simulink model "UG_model"  (R2024b)
settings: Solver=VariableStepAuto  StartTime=0.0  StopTime=500  FixedStep=0.0001  RelTol=1e-3
settings Model: Creator=yang1118  LastModifiedBy=leste
settings RTWCC: GPUComputeCapability=3.5

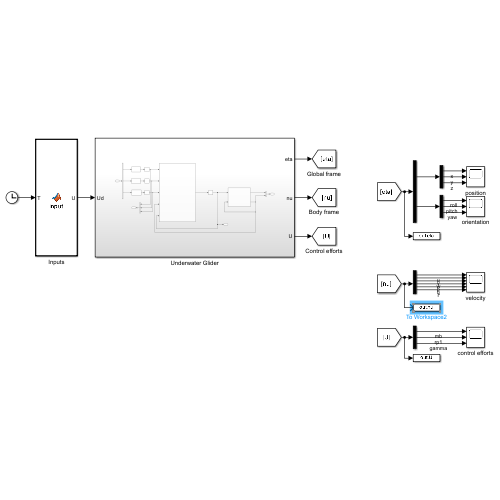
[thumbnail: Simulink's stored preview of the top-level diagram]
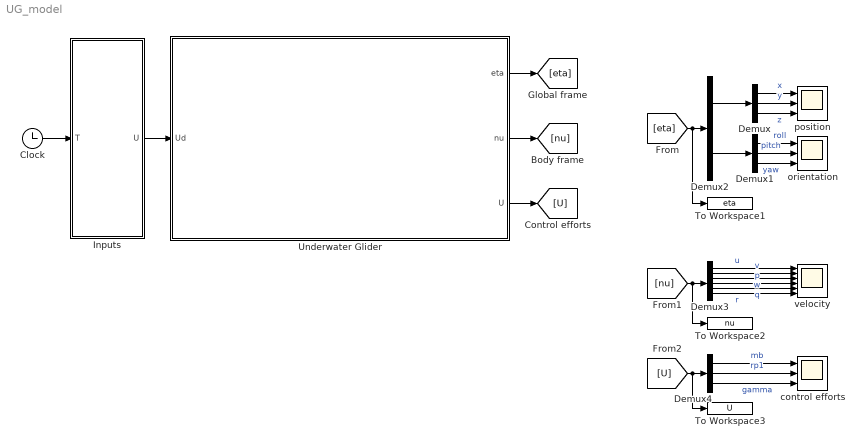
== system UG_model ==
  Clock : Clock
  Demux : Demux  Outputs=3
  Demux1 : Demux  Outputs=3
  Demux2 : Demux  Outputs=2
  Demux3 : Demux  Outputs=6
  Demux4 : Demux  Outputs=3
  Inputs : MATLAB Function  TreatAsAtomicUnit=on
  To Workspace1 : ToWorkspace  VariableName=eta  SampleTime=-1
      settings: Save2DSignal=2-D array (concatenate along first dimension)
  To Workspace2 : ToWorkspace  VariableName=nu  SampleTime=-1
      settings: Save2DSignal=2-D array (concatenate along first dimension)
  To Workspace3 : ToWorkspace  VariableName=U  SampleTime=-1
      settings: Save2DSignal=2-D array (concatenate along first dimension)
  Underwater Glider : Subsystem
  control efforts : Scope  NumInputPorts=3
  orientation : Scope  NumInputPorts=3
  position : Scope  NumInputPorts=3
  velocity : Scope  NumInputPorts=6
  wires:
  Clock/1 -> Inputs/1(T)
  Demux/1 -> position/1  "x"
  Demux/2 -> position/2  "y"
  Demux/3 -> position/3  "z"
  Demux1/1 -> orientation/1  "roll"
  Demux1/2 -> orientation/2  "pitch"
  Demux1/3 -> orientation/3  "yaw"
  Demux2/1 -> Demux/1
  Demux2/2 -> Demux1/1
  Demux3/5 -> velocity/5  "q"
  Demux3/6 -> velocity/6  "r"
  Demux3/2 -> velocity/2  "v"
  Demux3/1 -> velocity/1  "u"
  Demux3/3 -> velocity/3  "w"
  Demux3/4 -> velocity/4  "p"
  Inputs/1(U) -> Underwater Glider/1(Ud)
  Underwater Glider/1(eta) -> [eta]
  Underwater Glider/2(nu) -> [nu]
  Underwater Glider/3(U) -> [U]
  [eta] -> To Workspace1/1, Demux2/1
  [nu] -> To Workspace2/1, Demux3/1
  [U] -> To Workspace3/1, Demux4/1
  Demux4/1 -> control efforts/1  "mb"
  Demux4/2 -> control efforts/2  "rp1"
  Demux4/3 -> control efforts/3  "gamma"

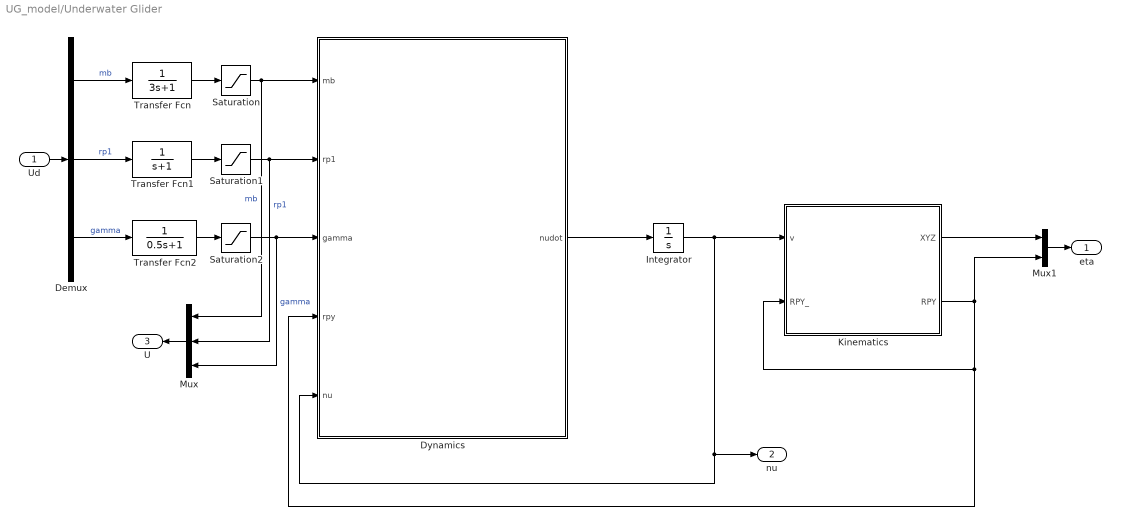
== system UG_model/Underwater Glider ==
  Ud : Inport
  Demux : Demux  Outputs=3
  Dynamics : MATLAB Function  TreatAsAtomicUnit=on
  Integrator : Integrator
  Kinematics : Subsystem
  Mux : Mux  Inputs=3
  Mux1 : Mux  Inputs=2
  Saturation : Saturate  UpperLimit=0.4  LowerLimit=-0.4
  Saturation1 : Saturate  UpperLimit=0.06  LowerLimit=-0.06
  Saturation2 : Saturate  UpperLimit=pi/2  LowerLimit=-pi/2
  Transfer Fcn : TransferFcn  Denominator=[3 1]
  Transfer Fcn1 : TransferFcn  Denominator=[1 1]
  Transfer Fcn2 : TransferFcn  Denominator=[0.5 1]
  eta : Outport
  nu : Outport  Port=2
  U : Outport  Port=3
  wires:
  Kinematics/2(RPY) -> Mux1/2, Kinematics/2(RPY_), Dynamics/4(rpy)
  Saturation/1 -> Mux/1, Dynamics/1(mb)  "mb"
  Saturation1/1 -> Dynamics/2(rp1), Mux/2  "rp1"
  Saturation2/1 -> Dynamics/3(gamma), Mux/3  "gamma"
  Dynamics/1(nudot) -> Integrator/1
  Integrator/1 -> nu/1, Dynamics/5(nu), Kinematics/1(v)
  Mux/1 -> U/1
  Transfer Fcn/1 -> Saturation/1
  Transfer Fcn1/1 -> Saturation1/1
  Transfer Fcn2/1 -> Saturation2/1
  Kinematics/1(XYZ) -> Mux1/1
  Mux1/1 -> eta/1
  Ud/1 -> Demux/1
  Demux/1 -> Transfer Fcn/1  "mb"
  Demux/2 -> Transfer Fcn1/1  "rp1"
  Demux/3 -> Transfer Fcn2/1  "gamma"

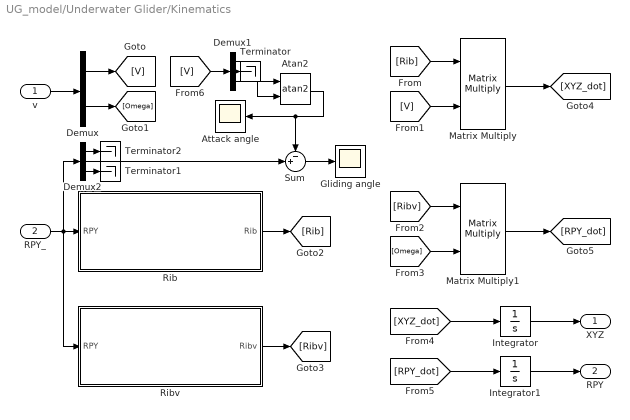
== system UG_model/Underwater Glider/Kinematics ==
  v : Inport  PortDimensions=[6,1]
  RPY_ : Inport  Port=2
  Atan2 : Trigonometry  Operator=atan2
  Attack angle : Scope
  Demux : Demux  Outputs=2
  Demux1 : Demux  Outputs=3
  Demux2 : Demux  Outputs=3
  Gliding angle : Scope
  Integrator : Integrator
  Integrator1 : Integrator
  Matrix Multiply : Product  Multiplication=Matrix(*)
  Matrix Multiply1 : Product  Multiplication=Matrix(*)
  Rib : Subsystem
  Ribv : Subsystem
  Sum : Sum  Inputs=-+|
  Terminator : Terminator
  Terminator1 : Terminator
  Terminator2 : Terminator
  XYZ : Outport
  RPY : Outport  Port=2
  wires:
  v/1 -> Demux/1
  Demux/1 -> [V]
  Demux/2 -> [Omega]
  RPY_/1 -> Demux2/1, Ribv/1(RPY), Rib/1(RPY)
  Rib/1(Rib) -> [Rib]
  Ribv/1(Ribv) -> [Ribv]
  [Rib] -> Matrix Multiply/1
  [V] -> Matrix Multiply/2
  Matrix Multiply/1 -> [XYZ_dot]
  [Ribv] -> Matrix Multiply1/1
  [Omega] -> Matrix Multiply1/2
  Matrix Multiply1/1 -> [RPY_dot]
  Integrator/1 -> XYZ/1
  Integrator1/1 -> RPY/1
  [XYZ_dot] -> Integrator/1
  [RPY_dot] -> Integrator1/1
  [V] -> Demux1/1
  Demux1/2 -> Terminator/1
  Demux1/3 -> Atan2/1
  Demux1/1 -> Atan2/2
  Demux2/3 -> Terminator1/1
  Demux2/1 -> Terminator2/1
  Sum/1 -> Gliding angle/1
  Demux2/2 -> Sum/2
  Atan2/1 -> Sum/1, Attack angle/1

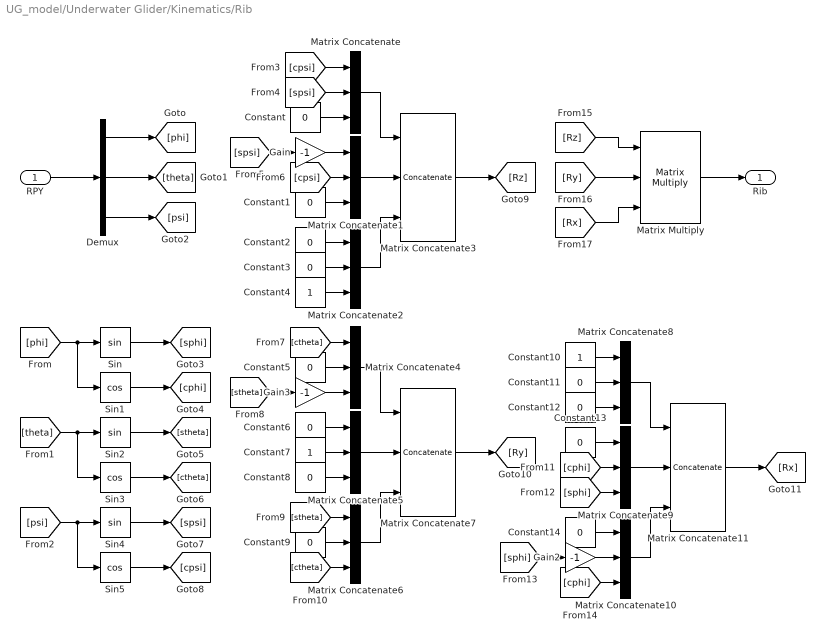
== system UG_model/Underwater Glider/Kinematics/Rib ==
  RPY : Inport  PortDimensions=[3,1]
  Constant{,1..3,5..6,8..9,11..14} (12 alike) : Constant  Value=0
  Constant10 : Constant
  Constant4 : Constant
  Constant7 : Constant
  Demux : Demux  Outputs=3
  Gain : Gain  Gain=-1
  Gain2 : Gain  Gain=-1
  Gain3 : Gain  Gain=-1
  Matrix Concatenate{,1..2,4..6,8..10} (9 alike) : Concatenate  NumInputs=3  ConcatenateDimension=2
  Matrix Concatenate11 : Concatenate  NumInputs=3  Mode=Multidimensional array  ConcatenateDimension=2
  Matrix Concatenate3 : Concatenate  NumInputs=3  Mode=Multidimensional array  ConcatenateDimension=2
  Matrix Concatenate7 : Concatenate  NumInputs=3  Mode=Multidimensional array  ConcatenateDimension=2
  Matrix Multiply : Product  Inputs=3  Multiplication=Matrix(*)
  Sin : Trigonometry
  Sin1 : Trigonometry  Operator=cos
  Sin2 : Trigonometry
  Sin3 : Trigonometry  Operator=cos
  Sin4 : Trigonometry
  Sin5 : Trigonometry  Operator=cos
  Rib : Outport  PortDimensions=[3,3]
  wires:
  Demux/3 -> [psi]
  Demux/1 -> [phi]
  Demux/2 -> [theta]
  RPY/1 -> Demux/1
  [phi] -> Sin1/1, Sin/1
  [theta] -> Sin2/1, Sin3/1
  [psi] -> Sin5/1, Sin4/1
  Sin/1 -> [sphi]
  Sin1/1 -> [cphi]
  Sin2/1 -> [stheta]
  Sin3/1 -> [ctheta]
  Sin4/1 -> [spsi]
  Sin5/1 -> [cpsi]
  [cpsi] -> Matrix Concatenate/1
  [spsi] -> Matrix Concatenate/2
  Constant/1 -> Matrix Concatenate/3
  Gain/1 -> Matrix Concatenate1/1
  [spsi] -> Gain/1
  [cpsi] -> Matrix Concatenate1/2
  Constant1/1 -> Matrix Concatenate1/3
  Constant2/1 -> Matrix Concatenate2/1
  Constant3/1 -> Matrix Concatenate2/2
  Constant4/1 -> Matrix Concatenate2/3
  Matrix Concatenate1/1 -> Matrix Concatenate3/2
  Matrix Concatenate/1 -> Matrix Concatenate3/1
  Matrix Concatenate2/1 -> Matrix Concatenate3/3
  Matrix Concatenate3/1 -> [Rz]
  Matrix Concatenate7/1 -> [Ry]
  Matrix Concatenate6/1 -> Matrix Concatenate7/3
  Matrix Concatenate4/1 -> Matrix Concatenate7/1
  Matrix Concatenate5/1 -> Matrix Concatenate7/2
  [ctheta] -> Matrix Concatenate4/1
  Constant5/1 -> Matrix Concatenate4/2
  [stheta] -> Gain3/1
  Constant6/1 -> Matrix Concatenate5/1
  Constant7/1 -> Matrix Concatenate5/2
  Constant8/1 -> Matrix Concatenate5/3
  Constant9/1 -> Matrix Concatenate6/2
  [ctheta] -> Matrix Concatenate6/3
  Matrix Concatenate9/1 -> Matrix Concatenate11/2
  Matrix Concatenate8/1 -> Matrix Concatenate11/1
  Matrix Concatenate10/1 -> Matrix Concatenate11/3
  Matrix Concatenate11/1 -> [Rx]
  Constant10/1 -> Matrix Concatenate8/1
  Constant11/1 -> Matrix Concatenate8/2
  Constant12/1 -> Matrix Concatenate8/3
  Constant13/1 -> Matrix Concatenate9/1
  [cphi] -> Matrix Concatenate9/2
  [sphi] -> Matrix Concatenate9/3
  Constant14/1 -> Matrix Concatenate10/1
  Gain2/1 -> Matrix Concatenate10/2
  [sphi] -> Gain2/1
  [cphi] -> Matrix Concatenate10/3
  [Ry] -> Matrix Multiply/2
  [Rx] -> Matrix Multiply/3
  [Rz] -> Matrix Multiply/1
  Matrix Multiply/1 -> Rib/1
  Gain3/1 -> Matrix Concatenate4/3
  [stheta] -> Matrix Concatenate6/1

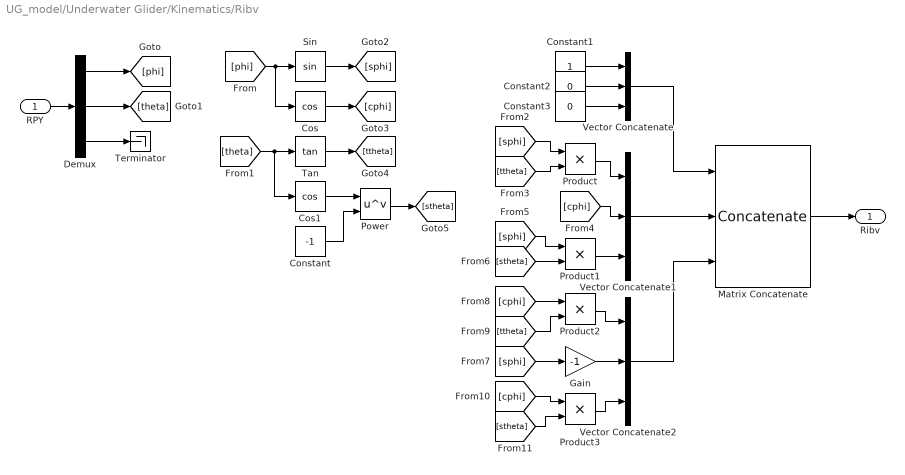
== system UG_model/Underwater Glider/Kinematics/Ribv ==
  RPY : Inport  PortDimensions=[3,1]
  Constant : Constant  Value=-1
  Constant1 : Constant
  Constant2 : Constant  Value=0
  Constant3 : Constant  Value=0
  Cos : Trigonometry  Operator=cos
  Cos1 : Trigonometry  Operator=cos
  Demux : Demux  Outputs=3
  Gain : Gain  Gain=-1
  Matrix Concatenate : Concatenate  NumInputs=3  Mode=Multidimensional array  ConcatenateDimension=2
  Power : Math  Operator=pow
  Product{,1..3} (4 alike) : Product
  Sin : Trigonometry
  Tan : Trigonometry  Operator=tan
  Terminator : Terminator
  Vector Concatenate : Concatenate  NumInputs=3
  Vector Concatenate1 : Concatenate  NumInputs=3
  Vector Concatenate2 : Concatenate  NumInputs=3
  Ribv : Outport  PortDimensions=[3,3]
  wires:
  RPY/1 -> Demux/1
  Demux/1 -> [phi]
  Demux/2 -> [theta]
  Demux/3 -> Terminator/1
  [phi] -> Cos/1, Sin/1
  Sin/1 -> [sphi]
  Cos/1 -> [cphi]
  [theta] -> Cos1/1, Tan/1
  Tan/1 -> [ttheta]
  Cos1/1 -> Power/1
  Constant/1 -> Power/2
  Power/1 -> [stheta]
  Constant1/1 -> Vector Concatenate/1
  Constant2/1 -> Vector Concatenate/2
  Constant3/1 -> Vector Concatenate/3
  Product/1 -> Vector Concatenate1/1
  [sphi] -> Product/1
  [ttheta] -> Product/2
  [cphi] -> Vector Concatenate1/2
  Product1/1 -> Vector Concatenate1/3
  [sphi] -> Product1/1
  [stheta] -> Product1/2
  Product2/1 -> Vector Concatenate2/1
  Product3/1 -> Vector Concatenate2/3
  Gain/1 -> Vector Concatenate2/2
  [sphi] -> Gain/1
  [cphi] -> Product2/1
  [ttheta] -> Product2/2
  [cphi] -> Product3/1
  [stheta] -> Product3/2
  Vector Concatenate1/1 -> Matrix Concatenate/2
  Vector Concatenate2/1 -> Matrix Concatenate/3
  Vector Concatenate/1 -> Matrix Concatenate/1
  Matrix Concatenate/1 -> Ribv/1

== matlab function UG_model/Underwater Glider/Dynamics ==
  data: mb input; nudot output; rp1 input; gamma input; rpy input; nu input
 function nudot  = fcn(mb, rp1, gamma, rpy, nu)

u = nu(1);
v = nu(2);
w = nu(3);
p = nu(4);
q = nu(5);
r = nu(6);

phi = rpy(1);
theta = rpy(2);
psi = rpy(3);

KD0 = 7.19;
KD = 386.29;
Kbeta = -115.65;
KL0 = -0.36;
KL = 440.99;
KMR = -58.27;
Kp = -19.83;
KM0 = 0.28;
KM = -65.84;
Kq = -205.64;
KMY = 34.10;
Kr = -389.30;

M = 54.28;
I = [0.6, 15.27, 15.32];
Mf1 = 1.48 + M;
Mf2 = 49.58 + M;
Mf3 = 65.92 + M;
If1 = 0.53 + I(1);
If2 = 7.88 + I(2);
If3 = 10.18 + I(3);

mp = 11;
g = 9.81;
Rp = 0.014;
Dglider = 0.22;
rho = 1000;
rb1 = mb/rho/(pi*(Dglider/2)^2);



udot = 1/Mf1 * (-KD0*u^2 + KL0*u*w - mb*g*sin(theta));

vdot = 1/Mf2 * ((Kbeta-KD0)*u*v + mb*g*sin(phi)*cos(theta) - r*u*Mf1);

wdot = 1/Mf3 * (-KL0*u^2 - (KL+KD0)*u*w + mb*g*cos(theta)*cos(phi));

pdot = 1/If1 * ((KMR-KM0)*u*v + Kp*p*u^2 - mp*Rp*g*cos(theta)*(cos(phi)*sin(gamma)+sin(phi)*cos(gamma)));

qdot = 1/If2 * ((Mf3-Mf1+KM)*u*w - mb*rb1*g*cos(theta)*cos(phi) - mp*g*(rp1*cos(theta)*cos(phi)+Rp*sin(theta)*cos(gamma)) + KM0*u^2 + Kq*q*u^2);

rdot = 1/If3 * (u*v*(Mf1-Mf2+KMY) + mb*rb1*g*sin(phi)*cos(theta) + mp*g*(rp1*sin(phi)*cos(theta)-Rp*sin(theta)*sin(gamma)) + Kr*r*u^2);


nudot = [udot;vdot;wdot;pdot;qdot;rdot];

== matlab function UG_model/Inputs ==
  data: T input; U output
function U = input(T)

t = mod(T,500);

if t <= 250
    mb = 0.4;
    rp1 = 0.06;
    gamma = pi/3;
else
    mb = -0.2;
    rp1 = -0.03;
    gamma = 0;
end

U = [mb,rp1,gamma]';
